simulink library "monroe_library"  (R2012b)
settings: Solver=ode45  StartTime=0.0  StopTime=10.0  RelTol=1e-3
values from neighbouring files (symbols this model uses):
  input_bit_width = ', num2str(input_bit_width))    [fft_direct_draw.m]
undefined symbols (not defined in the file or in its folder): gcbh, xlBlockLoadCallback
libraries: xbsIndex_r4 x1880, monroe_library x159, casper_library x13, xps_library x1
(part 36 of 43)

== system monroe_library/unscr_tail/reorder2 ==
  sync : Inport
  din0 : Inport  Port=2
  din1 : Inport  Port=3
  din2 : Inport  Port=4
  din3 : Inport  Port=5
  Concat2 : xbsIndex_r4/Concat  num_inputs=2  dbl_ovrd=off  block_type=concat
  Concat3 : xbsIndex_r4/Concat  num_inputs=2  dbl_ovrd=off  block_type=concat
  Constant1 : xbsIndex_r4/Constant  arith_type=Boolean  const=1  n_bits=1  bin_pt=0  explicit_period=on  period=1  equ=P=C  opselect=C  inp2=PCIN>>17  opr=+  inp1=P  carry=CIN  dbl_ovrd=off  block_type=constant
  Constant5 : xbsIndex_r4/Constant  arith_type=Boolean  const=1  n_bits=1  bin_pt=0  explicit_period=on  period=1  equ=P=C  opselect=C  inp2=PCIN>>17  opr=+  inp1=P  carry=CIN  dbl_ovrd=off  block_type=constant
  Constant7 : xbsIndex_r4/Constant  arith_type=Boolean  const=0  n_bits=1  bin_pt=0  explicit_period=on  period=1  equ=P=C  opselect=C  inp2=PCIN>>17  opr=+  inp1=P  carry=CIN  dbl_ovrd=off  block_type=constant
  Dual Port RAM1 : xbsIndex_r4/Dual Port RAM  depth=2^FFTSize  initVector=sin(pi*(0:15)/16)  distributed_mem=Block RAM  init_a=0  init_b=0  rst_a=off  rst_b=off  en_a=off  en_b=off  latency=bram_latency  write_mode_A=Read Before Write  write_mode_B=Read Before Write  dbl_ovrd=off  optimize=Area  use_rpm=on  block_type=dpram
  Dual Port RAM2 : xbsIndex_r4/Dual Port RAM  depth=2^FFTSize  initVector=sin(pi*(0:15)/16)  distributed_mem=Block RAM  init_a=0  init_b=0  rst_a=off  rst_b=off  en_a=off  en_b=off  latency=bram_latency  write_mode_A=Read Before Write  write_mode_B=Read Before Write  dbl_ovrd=off  optimize=Area  use_rpm=on  block_type=dpram
  addresser : Subsystem
  addresser1 : Subsystem
  delay_din{0..3} (4 alike) : xbsIndex_r4/Delay  en=off  latency=reorder_din_latency  dbl_ovrd=off  reg_retiming=off  block_type=delay
  pre_sync_delay1 : xbsIndex_r4/Delay  en=off  latency=reorder_din_latency  dbl_ovrd=off  reg_retiming=off  block_type=delay
  pre_sync_delay3 : xbsIndex_r4/Delay  en=off  latency=reorder_din_latency  dbl_ovrd=off  reg_retiming=off  block_type=delay
  sync_tree : Subsystem
  dout0 : Outport
  dout1 : Outport  Port=2
  dout2 : Outport  Port=3
  dout3 : Outport  Port=4
  wires:
  delay_din3/1 -> Dual Port RAM2/5
  delay_din2/1 -> Dual Port RAM2/2
  delay_din1/1 -> Dual Port RAM1/5
  delay_din0/1 -> Dual Port RAM1/2
  Constant1/1 -> Dual Port RAM2/3, Dual Port RAM2/6, Dual Port RAM1/3, Dual Port RAM1/6
  Dual Port RAM2/1 -> dout2/1
  Dual Port RAM2/2 -> dout3/1
  sync_tree/1(Out1) -> addresser/1(sync_in)
  sync_tree/2(Out2) -> addresser1/1(sync_in)
  sync/1 -> sync_tree/1(In1)
  addresser1/1(addr_out) -> pre_sync_delay1/1
  addresser/1(addr_out) -> pre_sync_delay3/1
  pre_sync_delay3/1 -> Concat2/2  "xlsub3_pre_sync_delay3_out1"
  pre_sync_delay1/1 -> Concat3/2
  din3/1 -> delay_din3/1
  din2/1 -> delay_din2/1
  din1/1 -> delay_din1/1
  din0/1 -> delay_din0/1
  Dual Port RAM1/1 -> dout0/1
  Dual Port RAM1/2 -> dout1/1
  Concat3/1 -> Dual Port RAM2/4, Dual Port RAM1/4
  Concat2/1 -> Dual Port RAM2/1, Dual Port RAM1/1
  Constant7/1 -> Concat3/1
  Constant5/1 -> Concat2/1

== system monroe_library/FFT_Biplex_4x/biplex_4x_unscr/dual_bit_reverse ==
  sync : Inport
  din0 : Inport  Port=2
  din1 : Inport  Port=3
  Concat1 : xbsIndex_r4/Concat  num_inputs=2  dbl_ovrd=off  block_type=concat
  Concat2 : xbsIndex_r4/Concat  num_inputs=2  dbl_ovrd=off  block_type=concat
  Constant : xbsIndex_r4/Constant  arith_type=Boolean  const=1  n_bits=1  bin_pt=0  explicit_period=on  period=1  equ=P=C  opselect=C  inp2=PCIN>>17  opr=+  inp1=P  carry=CIN  dbl_ovrd=off  block_type=constant
  Constant1 : xbsIndex_r4/Constant  arith_type=Boolean  const=0  n_bits=1  bin_pt=0  explicit_period=on  period=1  equ=P=C  opselect=C  inp2=PCIN>>17  opr=+  inp1=P  carry=CIN  dbl_ovrd=off  block_type=constant
  Constant5 : xbsIndex_r4/Constant  arith_type=Boolean  const=1  n_bits=1  bin_pt=0  explicit_period=on  period=1  equ=P=C  opselect=C  inp2=PCIN>>17  opr=+  inp1=P  carry=CIN  dbl_ovrd=off  block_type=constant
  Counter : xbsIndex_r4/Counter  cnt_type=Free Running  cnt_to=1023  operation=Up  start_count=0  cnt_by_val=1  arith_type=Unsigned  n_bits=10  bin_pt=0  load_pin=off  rst=on  en=off  explicit_period=on  period=1  dbl_ovrd=off  use_behavioral_HDL=off  implementation=Fabric  use_rpm=off  block_type=counter
  Counter1 : xbsIndex_r4/Counter  cnt_type=Free Running  cnt_to=1023  operation=Down  start_count=1023  cnt_by_val=1  arith_type=Unsigned  n_bits=10  bin_pt=0  load_pin=off  rst=on  en=off  explicit_period=on  period=1  dbl_ovrd=off  use_behavioral_HDL=off  implementation=Fabric  use_rpm=off  block_type=counter
  Dual Port RAM : xbsIndex_r4/Dual Port RAM  depth=1024  initVector=sin(pi*(0:15)/16)  distributed_mem=Block RAM  init_a=0  init_b=0  rst_a=off  rst_b=off  en_a=off  en_b=off  latency=2  write_mode_A=Read Before Write  write_mode_B=Read Before Write  dbl_ovrd=off  optimize=Area  use_rpm=on  block_type=dpram
  Inverter : xbsIndex_r4/Inverter  en=off  latency=0  dbl_ovrd=off  block_type=inv
  Mux : xbsIndex_r4/Mux  inputs=2  en=off  latency=0  precision=Full  arith_type=Unsigned  n_bits=16  bin_pt=14  quantization=Truncate  overflow=Wrap  dbl_ovrd=off  block_type=mux
  Mux1 : xbsIndex_r4/Mux  inputs=2  en=off  latency=0  precision=Full  arith_type=Unsigned  n_bits=16  bin_pt=14  quantization=Truncate  overflow=Wrap  dbl_ovrd=off  block_type=mux
  Slice1 : xbsIndex_r4/Slice  nbits=1  boolean_output=off  mode=Upper Bit Location + Width  bit1=0  base1=MSB of Input  bit0=0  base0=LSB of Input  dbl_ovrd=off  block_type=slice
  Slice2 : xbsIndex_r4/Slice  nbits=9  boolean_output=off  mode=Lower Bit Location + Width  bit1=0  base1=MSB of Input  bit0=0  base0=LSB of Input  dbl_ovrd=off  block_type=slice
  Slice3 : xbsIndex_r4/Slice  nbits=1  boolean_output=off  mode=Upper Bit Location + Width  bit1=0  base1=MSB of Input  bit0=0  base0=LSB of Input  dbl_ovrd=off  block_type=slice
  Slice4 : xbsIndex_r4/Slice  nbits=9  boolean_output=off  mode=Lower Bit Location + Width  bit1=0  base1=MSB of Input  bit0=0  base0=LSB of Input  dbl_ovrd=off  block_type=slice
  bit_reverse_1 : Subsystem
  bit_reverse_2 : Subsystem
  delay_din0 : xbsIndex_r4/Delay  en=off  latency=0  dbl_ovrd=off  reg_retiming=off  block_type=delay
  delay_din1 : xbsIndex_r4/Delay  en=off  latency=0  dbl_ovrd=off  reg_retiming=off  block_type=delay
  post_sync_delay : xbsIndex_r4/Delay  en=off  latency=2  dbl_ovrd=off  reg_retiming=off  block_type=delay
  post_sync_delay1 : xbsIndex_r4/Delay  en=off  latency=0  dbl_ovrd=off  reg_retiming=off  block_type=delay
  sync_delay_fast : monroe_library/sync_delay_fast  SystemSampleTime=-1  delay_len=512
  sync_out : Outport
  dout0 : Outport  Port=2
  dout1 : Outport  Port=3
  wires:
  Constant/1 -> Dual Port RAM/6, Dual Port RAM/3
  Counter/1 -> Slice2/1, Slice1/1
  Slice1/1 -> Mux1/1, Mux/1
  Slice2/1 -> bit_reverse_1/1(in), Mux1/2, Mux/2
  Counter1/1 -> Slice4/1, Slice3/1
  post_sync_delay1/1 -> sync_delay_fast/1, Counter1/1, Counter/1
  bit_reverse_2/1(out) -> Mux1/3
  Slice4/1 -> bit_reverse_2/1(in)  "xlsub3_Slice4_out1"
  bit_reverse_1/1(out) -> Mux/3
  sync_delay_fast/1 -> post_sync_delay/1
  sync/1 -> post_sync_delay1/1
  post_sync_delay/1 -> sync_out/1
  delay_din1/1 -> Dual Port RAM/5
  din1/1 -> delay_din1/1
  delay_din0/1 -> Dual Port RAM/2
  din0/1 -> delay_din0/1
  Slice3/1 -> Inverter/1
  Mux1/1 -> Concat1/2
  Mux/1 -> Concat2/2
  Dual Port RAM/2 -> dout1/1
  Dual Port RAM/1 -> dout0/1
  Concat1/1 -> Dual Port RAM/4
  Concat2/1 -> Dual Port RAM/1
  Constant5/1 -> Concat2/1
  Constant1/1 -> Concat1/1

== system monroe_library/FFT_Biplex_4x/biplex_muxsel_gen/coeff_gen10 ==
  sync : Inport
  Concat : xbsIndex_r4/Concat  num_inputs=2  dbl_ovrd=off  block_type=concat
  Concat1 : xbsIndex_r4/Concat  num_inputs=2  dbl_ovrd=off  block_type=concat
  Concat2 : xbsIndex_r4/Concat  num_inputs=2  dbl_ovrd=off  block_type=concat
  Constant : xbsIndex_r4/Constant  arith_type=Boolean  const=0  n_bits=16  bin_pt=14  explicit_period=on  period=1  equ=P=C  opselect=C  inp2=PCIN>>17  opr=+  inp1=P  carry=CIN  dbl_ovrd=off  block_type=constant
  Constant1 : xbsIndex_r4/Constant  arith_type=Boolean  const=1  n_bits=16  bin_pt=14  explicit_period=on  period=1  equ=P=C  opselect=C  inp2=PCIN>>17  opr=+  inp1=P  carry=CIN  dbl_ovrd=off  block_type=constant
  Constant3 : xbsIndex_r4/Constant  arith_type=Signed (2's comp)  const=0  n_bits=18  bin_pt=17  explicit_period=on  period=1  equ=P=C  opselect=C  inp2=PCIN>>17  opr=+  inp1=P  carry=CIN  dbl_ovrd=off  block_type=constant
  Constant4 : xbsIndex_r4/Constant  arith_type=Boolean  const=0  n_bits=16  bin_pt=14  explicit_period=on  period=1  equ=P=C  opselect=C  inp2=PCIN>>17  opr=+  inp1=P  carry=CIN  dbl_ovrd=off  block_type=constant
  Counter : xbsIndex_r4/Counter  cnt_type=Free Running  cnt_to=Inf  operation=Up  start_count=2  cnt_by_val=1  arith_type=Unsigned  n_bits=9  bin_pt=0  load_pin=off  rst=on  en=off  explicit_period=on  period=1  dbl_ovrd=off  use_behavioral_HDL=off  implementation=Fabric  block_type=counter
  Dual Port RAM4 : xbsIndex_r4/Dual Port RAM  depth=1024  initVector=[0 -1 -0.707106781186547 -0.707106781186548 -0.38268343236509 -0.923879532511287 -0.923879532511287 -0.38268343236509 -0.195090322016128 -0.98078528040323 -0.831469612302545 -0.555570233019602 -0.555570233019602 -0.831469612302545 -0.98078528040323 -0.195090322016129 -0.0980171403295606 -0.995184726672197 -0.773010453362737 -0.634393284163645 -0.471396736825998 -0.881921264348355 -0.956940335732209 -0.290284677254462 -0.290284677254462 -0.956940335732209 -0.881921264348355 -0.471396736825998 -0.634393284163645 -0.773010453362737 -0.995184726672197 -0.0980171403295608 -0.049067674327418 -0.998795456205172 -0.740951125354959 -0.671558954847019 -0.427555093430282 -0.903989293123443 -0.941544065183021 -0.33688985339222 -0.242980179903264 -0.970031253194544 -0.857728610000272 -0.514102744193222 -0.595699304492433 -0.803207531480645 -0.989176509964781 -0.146730474455362 -0.146730474455362 -0.989176509964781 -0.803207531480645 -0.595699304492433 -0.514102744193222 -0.857728610000272 -0.970031253194544 -0.242980179903264 -0.33688985339222 -0.941544065183021 -0.903989293123443 -0.427555093430282 -0.671558954847018 -0.740951125354959 -0.998795456205172 -0.049067674327418 -0.0245412285229123 -0.999698818696204 -0.724247082951467 -0.689540544737067 -0.40524131400499 -0.914209755703531 -0.932992798834739 -0.359895036534988 -0.21910124015687 -0.975702130038529 -0.844853565249707 -0.534997619887097 -0.575808191417845 -0.817584813151584 -0.985277642388941 -0.170961888760301 -0.122410675199216 -0.99247953459871 -0.788346427626606 -0.615231590580627 -0.492898192229784 -0.870086991108711 -0.96377606579544 -0.266712757474898 -0.313681740398892 -0.949528180593037 -0.893224301195515 -0.449611329654607 -0.653172842953777 -0.757208846506485 -0.99729045667869 -0.0735645635996677 -0.0735645635996674 -0.99729045667869 -0.757208846506485 -0.653172842953777 -0.449611329654607 -0.893224301195515 -0.949528180593037 -0.313681740398891 -0.266712757474898 -0.96377606579544 -0.870086991108711 -0.492898192229784 -0.615231590580627 -0.788346427626606 -0.99247953459871 -0.122410675199216 -0.170961888760301 -0.985277642388941 -0.817584813151584 -0.575808191417845 -0.534997619887097 -0.844853565249707 -0.975702130038529 -0.21910124015687 -0.359895036534988 -0.932992798834739 -0.914209755703531 -0.40524131400499 -0.689540544737067 -0.724247082951467 -0.999698818696204 -0.0245412285229123 -0.0122715382857199 -0.999924701839145 -0.715730825283819 -0.698376249408973 -0.393992040061048 -0.919113851690058 -0.928506080473216 -0.371317193951838 -0.207111376192219 -0.978317370719628 -0.838224705554838 -0.545324988422046 -0.565731810783613 -0.824589302785025 -0.983105487431216 -0.183039887955141 -0.110222207293883 -0.993906970002356 -0.780737228572094 -0.624859488142386 -0.482183772079123 -0.876070094195407 -0.960430519415566 -0.278519689385053 -0.302005949319228 -0.953306040354194 -0.887639620402854 -0.46053871095824 -0.643831542889791 -0.765167265622459 -0.996312612182778 -0.0857973123444402 -0.0613207363022086 -0.998118112900149 -0.749136394523459 -0.662415777590172 -0.438616238538528 -0.898674465693954 -0.945607325380521 -0.325310292162263 -0.254865659604515 -0.966976471044852 -0.863972856121587 -0.503538383725718 -0.605511041404326 -0.795836904608884 -0.99090263542778 -0.134580708507126 -0.158858143333861 -0.987301418157858 -0.810457198252595 -0.585797857456439 -0.524589682678469 -0.851355193105265 -0.97293995220556 -0.231058108280671 -0.348418680249435 -0.937339011912575 -0.909167983090522 -0.416429560097637 -0.680600997795453 -0.732654271672413 -0.99932238458835 -0.0368072229413588 -0.0368072229413588 -0.99932238458835 -0.732654271672413 -0.680600997795453 -0.416429560097637 -0.909167983090522 -0.937339011912575 -0.348418680249435 -0.231058108280671 -0.97293995220556 -0.851355193105265 -0.524589682678469 -0.585797857456439 -0.810457198252595 -0.987301418157858 -0.158858143333861 -0.134580708507126 -0.99090263542778 -0.795836904608884 -0.605511041404326 ...(+15102 chars)]  distributed_mem=Block RAM  init_a=0  init_b=0  rst_a=off  rst_b=off  en_a=off  en_b=off  latency=2  write_mode_A=No Read On Write  write_mode_B=No Read On Write  dbl_ovrd=off  optimize=Area  use_rpm=on  block_type=dpram
  Reinterpret : xbsIndex_r4/Reinterpret  force_arith_type=on  arith_type=Unsigned  force_bin_pt=on  bin_pt=0  block_type=reinterpret
      settings: infoedit="Changes signal type without altering the binary representation.   You can changed the signal between signed and unsigned, and relocate the binary point.<br><br>Hardware notes: In hardware this block costs nothing.<br><br>Example:  Suppose the input is 6 bits wide, signed, with 2 fractional bits, and the output is forced to unsigned with 0 fractional bits.  Then an input of -2.0 (1110.00 in binary 2's complement) becomes an output of 56 (111000 in binary)."
  Reinterpret1 : xbsIndex_r4/Reinterpret  force_arith_type=on  arith_type=Unsigned  force_bin_pt=on  bin_pt=0  block_type=reinterpret
      settings: infoedit="Changes signal type without altering the binary representation.   You can changed the signal between signed and unsigned, and relocate the binary point.<br><br>Hardware notes: In hardware this block costs nothing.<br><br>Example:  Suppose the input is 6 bits wide, signed, with 2 fractional bits, and the output is forced to unsigned with 0 fractional bits.  Then an input of -2.0 (1110.00 in binary 2's complement) becomes an output of 56 (111000 in binary)."
  count_slice : xbsIndex_r4/Slice  nbits=9  boolean_output=off  mode=Upper Bit Location + Width  bit1=0  base1=MSB of Input  bit0=0  base0=MSB of Input  dbl_ovrd=off  block_type=slice
  coeff : Outport
  wires:
  count_slice/1 -> Concat1/2, Concat/2
  Constant3/1 -> Dual Port RAM4/5, Dual Port RAM4/2
  Constant/1 -> Dual Port RAM4/6, Dual Port RAM4/3
  Reinterpret1/1 -> Concat2/2
  Dual Port RAM4/2 -> Reinterpret1/1  "xlsub2_Dual_Port_RAM4_out2"
  Reinterpret/1 -> Concat2/1
  Dual Port RAM4/1 -> Reinterpret/1  "xlsub2_Dual_Port_RAM4_out1"
  Concat1/1 -> Dual Port RAM4/4
  Concat/1 -> Dual Port RAM4/1
  Concat2/1 -> coeff/1
  Constant4/1 -> Concat1/1
  Constant1/1 -> Concat/1
  Counter/1 -> count_slice/1
  sync/1 -> Counter/1

== system monroe_library/FFT_Biplex_4x/biplex_muxsel_gen/coeff_gen3 ==
  sync : Inport
  Concat : xbsIndex_r4/Concat  num_inputs=2  dbl_ovrd=off  block_type=concat
  Concat1 : xbsIndex_r4/Concat  num_inputs=2  dbl_ovrd=off  block_type=concat
  Concat2 : xbsIndex_r4/Concat  num_inputs=2  dbl_ovrd=off  block_type=concat
  Constant : xbsIndex_r4/Constant  arith_type=Boolean  const=0  n_bits=16  bin_pt=14  explicit_period=on  period=1  equ=P=C  opselect=C  inp2=PCIN>>17  opr=+  inp1=P  carry=CIN  dbl_ovrd=off  block_type=constant
  Constant1 : xbsIndex_r4/Constant  arith_type=Boolean  const=1  n_bits=16  bin_pt=14  explicit_period=on  period=1  equ=P=C  opselect=C  inp2=PCIN>>17  opr=+  inp1=P  carry=CIN  dbl_ovrd=off  block_type=constant
  Constant3 : xbsIndex_r4/Constant  arith_type=Signed (2's comp)  const=0  n_bits=18  bin_pt=17  explicit_period=on  period=1  equ=P=C  opselect=C  inp2=PCIN>>17  opr=+  inp1=P  carry=CIN  dbl_ovrd=off  block_type=constant
  Constant4 : xbsIndex_r4/Constant  arith_type=Boolean  const=0  n_bits=16  bin_pt=14  explicit_period=on  period=1  equ=P=C  opselect=C  inp2=PCIN>>17  opr=+  inp1=P  carry=CIN  dbl_ovrd=off  block_type=constant
  Counter : xbsIndex_r4/Counter  cnt_type=Free Running  cnt_to=Inf  operation=Up  start_count=2  cnt_by_val=1  arith_type=Unsigned  n_bits=9  bin_pt=0  load_pin=off  rst=on  en=off  explicit_period=on  period=1  dbl_ovrd=off  use_behavioral_HDL=off  implementation=Fabric  block_type=counter
  Dual Port RAM4 : xbsIndex_r4/Dual Port RAM  depth=8  initVector=[0 -1 -0.707106781186547 -0.707106781186548 1 6.12323399573677e-017 0.707106781186548 -0.707106781186547]  distributed_mem=Distributed memory  init_a=0  init_b=0  rst_a=off  rst_b=off  en_a=off  en_b=off  latency=2  write_mode_A=No Read On Write  write_mode_B=No Read On Write  dbl_ovrd=off  optimize=Area  use_rpm=on  block_type=dpram
  Reinterpret : xbsIndex_r4/Reinterpret  force_arith_type=on  arith_type=Unsigned  force_bin_pt=on  bin_pt=0  block_type=reinterpret
      settings: infoedit="Changes signal type without altering the binary representation.   You can changed the signal between signed and unsigned, and relocate the binary point.<br><br>Hardware notes: In hardware this block costs nothing.<br><br>Example:  Suppose the input is 6 bits wide, signed, with 2 fractional bits, and the output is forced to unsigned with 0 fractional bits.  Then an input of -2.0 (1110.00 in binary 2's complement) becomes an output of 56 (111000 in binary)."
  Reinterpret1 : xbsIndex_r4/Reinterpret  force_arith_type=on  arith_type=Unsigned  force_bin_pt=on  bin_pt=0  block_type=reinterpret
      settings: infoedit="Changes signal type without altering the binary representation.   You can changed the signal between signed and unsigned, and relocate the binary point.<br><br>Hardware notes: In hardware this block costs nothing.<br><br>Example:  Suppose the input is 6 bits wide, signed, with 2 fractional bits, and the output is forced to unsigned with 0 fractional bits.  Then an input of -2.0 (1110.00 in binary 2's complement) becomes an output of 56 (111000 in binary)."
  count_slice : xbsIndex_r4/Slice  nbits=2  boolean_output=off  mode=Upper Bit Location + Width  bit1=0  base1=MSB of Input  bit0=0  base0=MSB of Input  dbl_ovrd=off  block_type=slice
  coeff : Outport
  wires:
  count_slice/1 -> Concat1/2, Concat/2
  Reinterpret1/1 -> Concat2/2
  Dual Port RAM4/2 -> Reinterpret1/1  "xlsub2_Dual_Port_RAM4_out2"
  Reinterpret/1 -> Concat2/1
  Dual Port RAM4/1 -> Reinterpret/1  "xlsub2_Dual_Port_RAM4_out1"
  Concat1/1 -> Dual Port RAM4/4
  Constant/1 -> Dual Port RAM4/3
  Constant3/1 -> Dual Port RAM4/2
  Concat/1 -> Dual Port RAM4/1
  Concat2/1 -> coeff/1
  Constant4/1 -> Concat1/1
  Constant1/1 -> Concat/1
  Counter/1 -> count_slice/1
  sync/1 -> Counter/1

== system monroe_library/FFT_Biplex_4x/biplex_muxsel_gen/coeff_gen4 ==
  sync : Inport
  Concat : xbsIndex_r4/Concat  num_inputs=2  dbl_ovrd=off  block_type=concat
  Concat1 : xbsIndex_r4/Concat  num_inputs=2  dbl_ovrd=off  block_type=concat
  Concat2 : xbsIndex_r4/Concat  num_inputs=2  dbl_ovrd=off  block_type=concat
  Constant : xbsIndex_r4/Constant  arith_type=Boolean  const=0  n_bits=16  bin_pt=14  explicit_period=on  period=1  equ=P=C  opselect=C  inp2=PCIN>>17  opr=+  inp1=P  carry=CIN  dbl_ovrd=off  block_type=constant
  Constant1 : xbsIndex_r4/Constant  arith_type=Boolean  const=1  n_bits=16  bin_pt=14  explicit_period=on  period=1  equ=P=C  opselect=C  inp2=PCIN>>17  opr=+  inp1=P  carry=CIN  dbl_ovrd=off  block_type=constant
  Constant3 : xbsIndex_r4/Constant  arith_type=Signed (2's comp)  const=0  n_bits=18  bin_pt=17  explicit_period=on  period=1  equ=P=C  opselect=C  inp2=PCIN>>17  opr=+  inp1=P  carry=CIN  dbl_ovrd=off  block_type=constant
  Constant4 : xbsIndex_r4/Constant  arith_type=Boolean  const=0  n_bits=16  bin_pt=14  explicit_period=on  period=1  equ=P=C  opselect=C  inp2=PCIN>>17  opr=+  inp1=P  carry=CIN  dbl_ovrd=off  block_type=constant
  Counter : xbsIndex_r4/Counter  cnt_type=Free Running  cnt_to=Inf  operation=Up  start_count=2  cnt_by_val=1  arith_type=Unsigned  n_bits=9  bin_pt=0  load_pin=off  rst=on  en=off  explicit_period=on  period=1  dbl_ovrd=off  use_behavioral_HDL=off  implementation=Fabric  block_type=counter
  Dual Port RAM4 : xbsIndex_r4/Dual Port RAM  depth=16  initVector=[0 -1 -0.707106781186547 -0.707106781186548 -0.38268343236509 -0.923879532511287 -0.923879532511287 -0.38268343236509 1 6.12323399573677e-017 0.707106781186548 -0.707106781186547 0.923879532511287 -0.38268343236509 0.38268343236509 -0.923879532511287]  distributed_mem=Distributed memory  init_a=0  init_b=0  rst_a=off  rst_b=off  en_a=off  en_b=off  latency=2  write_mode_A=No Read On Write  write_mode_B=No Read On Write  dbl_ovrd=off  optimize=Area  use_rpm=on  block_type=dpram
  Reinterpret : xbsIndex_r4/Reinterpret  force_arith_type=on  arith_type=Unsigned  force_bin_pt=on  bin_pt=0  block_type=reinterpret
      settings: infoedit="Changes signal type without altering the binary representation.   You can changed the signal between signed and unsigned, and relocate the binary point.<br><br>Hardware notes: In hardware this block costs nothing.<br><br>Example:  Suppose the input is 6 bits wide, signed, with 2 fractional bits, and the output is forced to unsigned with 0 fractional bits.  Then an input of -2.0 (1110.00 in binary 2's complement) becomes an output of 56 (111000 in binary)."
  Reinterpret1 : xbsIndex_r4/Reinterpret  force_arith_type=on  arith_type=Unsigned  force_bin_pt=on  bin_pt=0  block_type=reinterpret
      settings: infoedit="Changes signal type without altering the binary representation.   You can changed the signal between signed and unsigned, and relocate the binary point.<br><br>Hardware notes: In hardware this block costs nothing.<br><br>Example:  Suppose the input is 6 bits wide, signed, with 2 fractional bits, and the output is forced to unsigned with 0 fractional bits.  Then an input of -2.0 (1110.00 in binary 2's complement) becomes an output of 56 (111000 in binary)."
  count_slice : xbsIndex_r4/Slice  nbits=3  boolean_output=off  mode=Upper Bit Location + Width  bit1=0  base1=MSB of Input  bit0=0  base0=MSB of Input  dbl_ovrd=off  block_type=slice
  coeff : Outport
  wires:
  count_slice/1 -> Concat1/2, Concat/2
  Reinterpret1/1 -> Concat2/2
  Dual Port RAM4/2 -> Reinterpret1/1  "xlsub2_Dual_Port_RAM4_out2"
  Reinterpret/1 -> Concat2/1
  Dual Port RAM4/1 -> Reinterpret/1  "xlsub2_Dual_Port_RAM4_out1"
  Concat1/1 -> Dual Port RAM4/4
  Constant/1 -> Dual Port RAM4/3
  Constant3/1 -> Dual Port RAM4/2
  Concat/1 -> Dual Port RAM4/1
  Concat2/1 -> coeff/1
  Constant4/1 -> Concat1/1
  Constant1/1 -> Concat/1
  Counter/1 -> count_slice/1
  sync/1 -> Counter/1

== system monroe_library/FFT_Biplex_4x/biplex_muxsel_gen/coeff_gen5 ==
  sync : Inport
  Concat : xbsIndex_r4/Concat  num_inputs=2  dbl_ovrd=off  block_type=concat
  Concat1 : xbsIndex_r4/Concat  num_inputs=2  dbl_ovrd=off  block_type=concat
  Concat2 : xbsIndex_r4/Concat  num_inputs=2  dbl_ovrd=off  block_type=concat
  Constant : xbsIndex_r4/Constant  arith_type=Boolean  const=0  n_bits=16  bin_pt=14  explicit_period=on  period=1  equ=P=C  opselect=C  inp2=PCIN>>17  opr=+  inp1=P  carry=CIN  dbl_ovrd=off  block_type=constant
  Constant1 : xbsIndex_r4/Constant  arith_type=Boolean  const=1  n_bits=16  bin_pt=14  explicit_period=on  period=1  equ=P=C  opselect=C  inp2=PCIN>>17  opr=+  inp1=P  carry=CIN  dbl_ovrd=off  block_type=constant
  Constant3 : xbsIndex_r4/Constant  arith_type=Signed (2's comp)  const=0  n_bits=18  bin_pt=17  explicit_period=on  period=1  equ=P=C  opselect=C  inp2=PCIN>>17  opr=+  inp1=P  carry=CIN  dbl_ovrd=off  block_type=constant
  Constant4 : xbsIndex_r4/Constant  arith_type=Boolean  const=0  n_bits=16  bin_pt=14  explicit_period=on  period=1  equ=P=C  opselect=C  inp2=PCIN>>17  opr=+  inp1=P  carry=CIN  dbl_ovrd=off  block_type=constant
  Counter : xbsIndex_r4/Counter  cnt_type=Free Running  cnt_to=Inf  operation=Up  start_count=2  cnt_by_val=1  arith_type=Unsigned  n_bits=9  bin_pt=0  load_pin=off  rst=on  en=off  explicit_period=on  period=1  dbl_ovrd=off  use_behavioral_HDL=off  implementation=Fabric  block_type=counter
  Dual Port RAM4 : xbsIndex_r4/Dual Port RAM  depth=32  initVector=[0 -1 -0.707106781186547 -0.707106781186548 -0.38268343236509 -0.923879532511287 -0.923879532511287 -0.38268343236509 -0.195090322016128 -0.98078528040323 -0.831469612302545 -0.555570233019602 -0.555570233019602 -0.831469612302545 -0.98078528040323 -0.195090322016129 1 6.12323399573677e-017 0.707106781186548 -0.707106781186547 0.923879532511287 -0.38268343236509 0.38268343236509 -0.923879532511287 0.98078528040323 -0.195090322016128 0.555570233019602 -0.831469612302545 0.831469612302545 -0.555570233019602 0.195090322016128 -0.98078528040323]  distributed_mem=Block RAM  init_a=0  init_b=0  rst_a=off  rst_b=off  en_a=off  en_b=off  latency=2  write_mode_A=No Read On Write  write_mode_B=No Read On Write  dbl_ovrd=off  optimize=Area  use_rpm=on  block_type=dpram
  Reinterpret : xbsIndex_r4/Reinterpret  force_arith_type=on  arith_type=Unsigned  force_bin_pt=on  bin_pt=0  block_type=reinterpret
      settings: infoedit="Changes signal type without altering the binary representation.   You can changed the signal between signed and unsigned, and relocate the binary point.<br><br>Hardware notes: In hardware this block costs nothing.<br><br>Example:  Suppose the input is 6 bits wide, signed, with 2 fractional bits, and the output is forced to unsigned with 0 fractional bits.  Then an input of -2.0 (1110.00 in binary 2's complement) becomes an output of 56 (111000 in binary)."
  Reinterpret1 : xbsIndex_r4/Reinterpret  force_arith_type=on  arith_type=Unsigned  force_bin_pt=on  bin_pt=0  block_type=reinterpret
      settings: infoedit="Changes signal type without altering the binary representation.   You can changed the signal between signed and unsigned, and relocate the binary point.<br><br>Hardware notes: In hardware this block costs nothing.<br><br>Example:  Suppose the input is 6 bits wide, signed, with 2 fractional bits, and the output is forced to unsigned with 0 fractional bits.  Then an input of -2.0 (1110.00 in binary 2's complement) becomes an output of 56 (111000 in binary)."
  count_slice : xbsIndex_r4/Slice  nbits=4  boolean_output=off  mode=Upper Bit Location + Width  bit1=0  base1=MSB of Input  bit0=0  base0=MSB of Input  dbl_ovrd=off  block_type=slice
  coeff : Outport
  wires:
  count_slice/1 -> Concat1/2, Concat/2
  Constant3/1 -> Dual Port RAM4/5, Dual Port RAM4/2
  Constant/1 -> Dual Port RAM4/6, Dual Port RAM4/3
  Reinterpret1/1 -> Concat2/2
  Dual Port RAM4/2 -> Reinterpret1/1  "xlsub2_Dual_Port_RAM4_out2"
  Reinterpret/1 -> Concat2/1
  Dual Port RAM4/1 -> Reinterpret/1  "xlsub2_Dual_Port_RAM4_out1"
  Concat1/1 -> Dual Port RAM4/4
  Concat/1 -> Dual Port RAM4/1
  Concat2/1 -> coeff/1
  Constant4/1 -> Concat1/1
  Constant1/1 -> Concat/1
  Counter/1 -> count_slice/1
  sync/1 -> Counter/1

== system monroe_library/FFT_Biplex_4x/biplex_muxsel_gen/coeff_gen6 ==
  sync : Inport
  Concat : xbsIndex_r4/Concat  num_inputs=2  dbl_ovrd=off  block_type=concat
  Concat1 : xbsIndex_r4/Concat  num_inputs=2  dbl_ovrd=off  block_type=concat
  Concat2 : xbsIndex_r4/Concat  num_inputs=2  dbl_ovrd=off  block_type=concat
  Constant : xbsIndex_r4/Constant  arith_type=Boolean  const=0  n_bits=16  bin_pt=14  explicit_period=on  period=1  equ=P=C  opselect=C  inp2=PCIN>>17  opr=+  inp1=P  carry=CIN  dbl_ovrd=off  block_type=constant
  Constant1 : xbsIndex_r4/Constant  arith_type=Boolean  const=1  n_bits=16  bin_pt=14  explicit_period=on  period=1  equ=P=C  opselect=C  inp2=PCIN>>17  opr=+  inp1=P  carry=CIN  dbl_ovrd=off  block_type=constant
  Constant3 : xbsIndex_r4/Constant  arith_type=Signed (2's comp)  const=0  n_bits=18  bin_pt=17  explicit_period=on  period=1  equ=P=C  opselect=C  inp2=PCIN>>17  opr=+  inp1=P  carry=CIN  dbl_ovrd=off  block_type=constant
  Constant4 : xbsIndex_r4/Constant  arith_type=Boolean  const=0  n_bits=16  bin_pt=14  explicit_period=on  period=1  equ=P=C  opselect=C  inp2=PCIN>>17  opr=+  inp1=P  carry=CIN  dbl_ovrd=off  block_type=constant
  Counter : xbsIndex_r4/Counter  cnt_type=Free Running  cnt_to=Inf  operation=Up  start_count=2  cnt_by_val=1  arith_type=Unsigned  n_bits=9  bin_pt=0  load_pin=off  rst=on  en=off  explicit_period=on  period=1  dbl_ovrd=off  use_behavioral_HDL=off  implementation=Fabric  block_type=counter
  Dual Port RAM4 : xbsIndex_r4/Dual Port RAM  depth=64  initVector=[0 -1 -0.707106781186547 -0.707106781186548 -0.38268343236509 -0.923879532511287 -0.923879532511287 -0.38268343236509 -0.195090322016128 -0.98078528040323 -0.831469612302545 -0.555570233019602 -0.555570233019602 -0.831469612302545 -0.98078528040323 -0.195090322016129 -0.0980171403295606 -0.995184726672197 -0.773010453362737 -0.634393284163645 -0.471396736825998 -0.881921264348355 -0.956940335732209 -0.290284677254462 -0.290284677254462 -0.956940335732209 -0.881921264348355 -0.471396736825998 -0.634393284163645 -0.773010453362737 -0.995184726672197 -0.0980171403295608 1 6.12323399573677e-017 0.707106781186548 -0.707106781186547 0.923879532511287 -0.38268343236509 0.38268343236509 -0.923879532511287 0.98078528040323 -0.195090322016128 0.555570233019602 -0.831469612302545 0.831469612302545 -0.555570233019602 0.195090322016128 -0.98078528040323 0.995184726672197 -0.0980171403295606 0.634393284163645 -0.773010453362737 0.881921264348355 -0.471396736825998 0.290284677254462 -0.956940335732209 0.956940335732209 -0.290284677254462 0.471396736825998 -0.881921264348355 0.773010453362737 -0.634393284163645 0.0980171403295608 -0.995184726672197]  distributed_mem=Block RAM  init_a=0  init_b=0  rst_a=off  rst_b=off  en_a=off  en_b=off  latency=2  write_mode_A=No Read On Write  write_mode_B=No Read On Write  dbl_ovrd=off  optimize=Area  use_rpm=on  block_type=dpram
  Reinterpret : xbsIndex_r4/Reinterpret  force_arith_type=on  arith_type=Unsigned  force_bin_pt=on  bin_pt=0  block_type=reinterpret
      settings: infoedit="Changes signal type without altering the binary representation.   You can changed the signal between signed and unsigned, and relocate the binary point.<br><br>Hardware notes: In hardware this block costs nothing.<br><br>Example:  Suppose the input is 6 bits wide, signed, with 2 fractional bits, and the output is forced to unsigned with 0 fractional bits.  Then an input of -2.0 (1110.00 in binary 2's complement) becomes an output of 56 (111000 in binary)."
  Reinterpret1 : xbsIndex_r4/Reinterpret  force_arith_type=on  arith_type=Unsigned  force_bin_pt=on  bin_pt=0  block_type=reinterpret
      settings: infoedit="Changes signal type without altering the binary representation.   You can changed the signal between signed and unsigned, and relocate the binary point.<br><br>Hardware notes: In hardware this block costs nothing.<br><br>Example:  Suppose the input is 6 bits wide, signed, with 2 fractional bits, and the output is forced to unsigned with 0 fractional bits.  Then an input of -2.0 (1110.00 in binary 2's complement) becomes an output of 56 (111000 in binary)."
  count_slice : xbsIndex_r4/Slice  nbits=5  boolean_output=off  mode=Upper Bit Location + Width  bit1=0  base1=MSB of Input  bit0=0  base0=MSB of Input  dbl_ovrd=off  block_type=slice
  coeff : Outport
  wires:
  count_slice/1 -> Concat1/2, Concat/2
  Constant3/1 -> Dual Port RAM4/5, Dual Port RAM4/2
  Constant/1 -> Dual Port RAM4/6, Dual Port RAM4/3
  Reinterpret1/1 -> Concat2/2
  Dual Port RAM4/2 -> Reinterpret1/1  "xlsub2_Dual_Port_RAM4_out2"
  Reinterpret/1 -> Concat2/1
  Dual Port RAM4/1 -> Reinterpret/1  "xlsub2_Dual_Port_RAM4_out1"
  Concat1/1 -> Dual Port RAM4/4
  Concat/1 -> Dual Port RAM4/1
  Concat2/1 -> coeff/1
  Constant4/1 -> Concat1/1
  Constant1/1 -> Concat/1
  Counter/1 -> count_slice/1
  sync/1 -> Counter/1
